simulink model "CAMFC2_01_WMR01"  (R2017b)
settings: Solver=ode45  StartTime=0.0  StopTime=150  RelTol=1e-3  EnableMultiTasking=on
InitFcn:
  | constant_CAMFC2_01_WMR01
values from neighbouring files (symbols this model uses):
  alpha = 0.1    [constant_CAMFC2_01_WMR01.m]    (also in constant_CAMFC2_04_Comp.m = 0.01; constant_CAMFC2_04_Quad_03.m; constant_CAMFC2_04_Simple.m = 0.01; constant_CAMFC2_04_Simple_DoubleIntegrator.m = 0.01)
  AN = [     0 1 0 0 ... (first row only)    [constant_CAMFC2_01_WMR01.m]    (also in constant_CAMFC2_04_Comp.m = [     0 1 0 0 1; constant_CAMFC2_04_Quad_03.m; constant_CAMFC2_04_Simple.m; constant_CAMFC2_04_Simple_DoubleIntegrator.m)
  B = eye(n)    [constant_CAMFC2_01_WMR01.m]    (also in constant_CAMFC2_04_Quad_03.m; constant_CAMFC2_Quad_New_02.m)
  B_pseudo_inverse = ((B'*B)^(-1))*B'    [constant_CAMFC2_01_WMR01.m]    (also in constant_CAMFC2_Quad_New_02.m)
  BN = [     1 0 0 0 ... (first row only)    [constant_CAMFC2_01_WMR01.m]    (also in constant_CAMFC2_04_Comp.m = [     0 0 0 0 0; constant_CAMFC2_04_Quad_03.m; constant_CAMFC2_04_Simple.m; constant_CAMFC2_04_Simple_DoubleIntegrator.m)
  chi = [0 0 0 0 ... (first row only)    [constant_CAMFC2_01_WMR01.m]    (also in constant_CAMFC2_04_Comp.m = X_m*ones(n0,1); constant_CAMFC2_04_Quad_03.m = X_m*ones(n0,1); constant_CAMFC2_04_Simple.m = X_m*ones(n0,1); constant_CAMFC2_04_Simple_DoubleIntegrator.m = X_m*ones(n0,1))
  Cv = 0.1    [constant_CAMFC2_01_WMR01.m]
  Cw = 0.1    [constant_CAMFC2_01_WMR01.m]
  epsilon_struct = struct('data',epsilon_InitVal)    [constant_CAMFC2_01_WMR01.m]    (also in constant_CAMFC2_04_Comp.m; constant_CAMFC2_04_Quad_03.m; constant_CAMFC2_04_Simple.m; constant_CAMFC2_04_Simple_DoubleIntegrator.m)
  gama1 = 1e4*diag([1e-6*ones(2,1);1e0*ones(2,1)])    [constant_CAMFC2_01_WMR01.m]    (also in constant_CAMFC2_04_Comp.m = 1e+3*diag([1e-6;1e-0]); constant_CAMFC2_04_Quad_03.m = 1e+2*diag(1e-0*ones(n0,1)); constant_CAMFC2_04_Simple.m = 1e+2*diag([1e-0;1e-0]); constant_CAMFC2_04_Simple_Formation.m = 1e+2*diag([1e-0;1e-0]))
  gama2 = 1e-2*diag([1e-6*ones(2,1);1e0*ones(2,1)])    [constant_CAMFC2_01_WMR01.m]    (also in constant_CAMFC2_04_Comp.m = 1e+0*diag([1e-6;1e-0]); constant_CAMFC2_04_Quad_03.m = 1e+0*diag(1e-0*ones(n0,1)); constant_CAMFC2_04_Simple.m = 1e+1*diag([1e-0;1e-0]); constant_CAMFC2_04_Simple_Formation.m = 1e+1*diag([1e-0;1e-0]))
  H = L + BN    [constant_CAMFC2_01_WMR01.m]    (also in constant_CAMFC2_04_Comp.m; constant_CAMFC2_04_Quad_03.m; constant_CAMFC2_04_Simple.m; constant_CAMFC2_04_Simple_DoubleIntegrator.m)
  J = 0.01    [constant_CAMFC2_01_WMR01.m]    (also in constant_CAMFC2_04_Quad_03.m = 1.0e-3 * diag([1 1 2],0); constant_CAMFC2_Quad_New_02.m = 1.2416e-3 * diag([1 1 2],0))
  K = 1e-2*eye(n)    [constant_CAMFC2_01_WMR01.m]    (also in constant_CAMFC2_Quad_New_02.m = 1e+1*eye(n))
  k1 = 1    [constant_CAMFC2_01_WMR01.m]    (also in constant_CAMFC2_04_Comp.m; constant_CAMFC2_04_Quad_03.m = 50; constant_CAMFC2_04_Simple.m; constant_CAMFC2_04_Simple_DoubleIntegrator.m)
  k2 = 1    [constant_CAMFC2_01_WMR01.m]    (also in constant_CAMFC2_04_Comp.m; constant_CAMFC2_04_Quad_03.m; constant_CAMFC2_04_Simple.m; constant_CAMFC2_04_Simple_DoubleIntegrator.m)
  L0 = 0.1    [constant_CAMFC2_01_WMR01.m]
  M = 1    [constant_CAMFC2_01_WMR01.m]    (also in constant_CAMFC2_04_Quad_03.m = 2; constant_CAMFC2_Quad_New_02.m = 2)
  N = 4    [constant_CAMFC2_01_WMR01.m]    (also in constant_CAMFC2_04_Comp.m = 5; constant_CAMFC2_04_Quad_03.m; constant_CAMFC2_04_Simple.m; constant_CAMFC2_04_Simple_DoubleIntegrator.m)
  n = 4    [constant_CAMFC2_01_WMR01.m]    (also in constant_CAMFC2_04_Comp.m = 2; constant_CAMFC2_04_Quad_03.m = 6; constant_CAMFC2_04_Simple.m = 2; constant_CAMFC2_04_Simple_DoubleIntegrator.m = 2)
  n0 = 2    [constant_CAMFC2_01_WMR01.m]    (also in constant_CAMFC2_04_Comp.m = 1; constant_CAMFC2_04_Quad_03.m = 3; constant_CAMFC2_04_Simple.m; constant_CAMFC2_04_Simple_DoubleIntegrator.m = 1)
  Observer_Gain = 100    [constant_CAMFC2_01_WMR01.m]    (also in constant_CAMFC2_04_Comp.m = 10; constant_CAMFC2_04_Quad_03.m = 1; constant_CAMFC2_04_Simple.m; constant_CAMFC2_04_Simple_DoubleIntegrator.m)
  Observer_Gain1 = 100    [constant_CAMFC2_01_WMR01.m]    (also in constant_CAMFC2_04_Comp.m = 10; constant_CAMFC2_04_Quad_03.m = 1; constant_CAMFC2_04_Simple.m; constant_CAMFC2_04_Simple_DoubleIntegrator.m)
  P_struct = struct('data',P_InitVal)    [constant_CAMFC2_01_WMR01.m]    (also in constant_CAMFC2_04_Comp.m; constant_CAMFC2_04_Quad_03.m; constant_CAMFC2_04_Simple.m; constant_CAMFC2_04_Simple_DoubleIntegrator.m)
  Q = 1e-0*eye(n)    [constant_CAMFC2_01_WMR01.m]    (also in constant_CAMFC2_04_Comp.m = 1.0e+2*eye(n); constant_CAMFC2_04_Quad_03.m = 1e-0*eye(n0); constant_CAMFC2_04_Simple.m = 1.0e+1*eye(n); constant_CAMFC2_04_Simple_Formation.m = 1.0e+1*eye(n))
  R = 1e-0*eye(n)    [constant_CAMFC2_01_WMR01.m]    (also in constant_CAMFC2_04_Quad_03.m; constant_CAMFC2_Quad_New_02.m = 1e+0*eye(n))
  R0 = 0.1    [constant_CAMFC2_01_WMR01.m]
  rho1 = 1e-1    (= 0.1)    [constant_CAMFC2_01_WMR01.m]    (also in constant_CAMFC2_04_Comp.m = 1; constant_CAMFC2_04_Quad_03.m = 1; constant_CAMFC2_04_Simple.m = 1; constant_CAMFC2_04_Simple_DoubleIntegrator.m = 1)
  rho2 = 1e-3    (= 0.001)    [constant_CAMFC2_01_WMR01.m]    (also in constant_CAMFC2_04_Comp.m = 1; constant_CAMFC2_04_Quad_03.m = 1; constant_CAMFC2_04_Simple.m = 1; constant_CAMFC2_04_Simple_DoubleIntegrator.m = 10)
  T_struct = struct('data',T_InitVal)    [constant_CAMFC2_01_WMR01.m]    (also in constant_CAMFC2_04_Comp.m; constant_CAMFC2_04_Quad_03.m; constant_CAMFC2_04_Simple.m; constant_CAMFC2_04_Simple_DoubleIntegrator.m)
  Thresh = 1e-4    (= 0.0001)    [constant_CAMFC2_01_WMR01.m]
  U_dot0_M = U_dot0_m*ones(n,1)    [constant_CAMFC2_01_WMR01.m]    (also in constant_CAMFC2_Quad_New_02.m = U_dot0_m*ones(n0,1))
  Upsilon_M = Upsilon_m*ones(n,1)    [constant_CAMFC2_01_WMR01.m]    (also in constant_CAMFC2_04_Comp.m; constant_CAMFC2_04_Quad_03.m = Upsilon_m*ones(n0,1); constant_CAMFC2_04_Simple.m; constant_CAMFC2_04_Simple_DoubleIntegrator.m)
libraries: simulink x1
(part 1 of 2)
settings Model: SimulationMode=rapid-accelerator  ExtModeTrigDuration=100  Creator=hp  LastModifiedBy=ali.safaei
settings DataIOCC: LimitDataPoints=on  SaveFinalState=on  SaveFormat=StructureWithTime  SaveOutput=off  SaveState=on  StateSaveName=tmp_raccel_xout  SignalLoggingName=tmp_raccel_logsout
settings OptimizationCC: EfficientMapNaN2IntZero=off  LifeSpan=inf
settings DebuggingCC: UnderspecifiedInitializationDetection=Classic  MergeDetectMultiDrivingBlocksExec=none  SFUnexpectedBacktrackingDiag=warning  SFNoUnconditionalDefaultTransitionDiag=warning  SFExecutionAtInitializationDiag=none
settings HardwareCC: ProdBitPerPointer=32  ProdBitPerSizeT=32  ProdBitPerPtrDiffT=32  ProdLargestAtomicFloat=None  ProdIntDivRoundTo=Undefined  ProdEndianess=Unspecified  ProdWordSize=32  ProdHWDeviceType=32-bit Generic  TargetBitPerPointer=64  TargetBitPerSizeT=64  TargetBitPerPtrDiffT=64  TargetLongLongMode=on  TargetIntDivRoundTo=Zero  TargetEndianess=LittleEndian  TargetWordSize=64  TargetHWDeviceType=MATLAB Host  ProdEqTarget=off
settings ModelReferenceCC: PropagateSignalLabelsOutOfModel=off
settings RTWCC: SystemTargetFile=raccel.tlc  TemplateMakefile=raccel_default_tmf  RTWVerbose=off  RTWUseSimCustomCode=on
settings CodeAppCC: GenerateComments=off  MaxIdLength=128  MangleLength=10  SimulinkBlockComments=off
settings RaccelTargetCC: GeneratePreprocessorConditionals=Use local settings  MultiInstanceERTCode=off  ExtModeMexArgs='', 0, 54523  ENABLE_SLEXEC_SSBRIDGE=0  RTWCAPIParams=on
settings ConfigComp: CovMetricSettings=dw  CovHtmlReporting=on  CovSaveCumulativeToWorkspaceVar=on  CovSaveSingleToWorkspaceVar=on  CovExternalEMLEnable=off

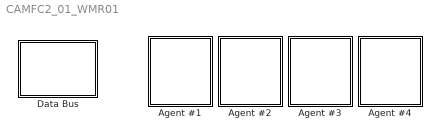
== system CAMFC2_01_WMR01 ==
  Agent #1 : Subsystem
  Agent #2 : Subsystem
  Agent #3 : Subsystem
  Agent #4 : Subsystem
  "Data Bus " : Subsystem

== system CAMFC2_01_WMR01/Agent #1 ==
  Agent # : Constant
  Controller interpreter : MATLAB Function  TreatAsAtomicUnit=on
  Decenteralized Cooperaive Controller #1 : Subsystem
  WMR Plant-01 : Subsystem
  tag scope: x1=global
  wires:
  Decenteralized Cooperaive Controller #1/1(U1) -> Controller interpreter/1(U)
  Agent #/1 -> Decenteralized Cooperaive Controller #1/1(Agent #)
  WMR Plant-01/1(Y) -> [x1]
  Controller interpreter/1(u) -> WMR Plant-01/1(U)

== system CAMFC2_01_WMR01/Agent #2 ==
  Agent # : Constant  Value=2
  Controller interpreter : MATLAB Function  TreatAsAtomicUnit=on
  Decenteralized Cooperaive Controller #2 : Subsystem
  WMR Plant-02 : Subsystem
  tag scope: x2=global
  wires:
  Agent #/1 -> Decenteralized Cooperaive Controller #2/1(Agent #)
  WMR Plant-02/1(Y) -> [x2]
  Decenteralized Cooperaive Controller #2/1(U2) -> Controller interpreter/1(U)
  Controller interpreter/1(u) -> WMR Plant-02/1(U)

== system CAMFC2_01_WMR01/Agent #3 ==
  Agent # : Constant  Value=3
  Controller interpreter : MATLAB Function  TreatAsAtomicUnit=on
  Decenteralized Cooperaive Controller #3 : Subsystem
  WMR Plant-03 : Subsystem
  tag scope: x3=global
  wires:
  Agent #/1 -> Decenteralized Cooperaive Controller #3/1(Agent #)
  WMR Plant-03/1(Y) -> [x3]
  Decenteralized Cooperaive Controller #3/1(U3) -> Controller interpreter/1(U)
  Controller interpreter/1(u) -> WMR Plant-03/1(U)

== system CAMFC2_01_WMR01/Agent #4 ==
  Agent # : Constant  Value=4
  Controller interpreter : MATLAB Function  TreatAsAtomicUnit=on
  Decenteralized Cooperaive Controller #4 : Subsystem
  WMR Plant-04 : Subsystem
  tag scope: x4=global
  wires:
  WMR Plant-04/1(Y) -> [x4]
  Agent #/1 -> Decenteralized Cooperaive Controller #4/1(Agent #)
  Decenteralized Cooperaive Controller #4/1(U4) -> Controller interpreter/1(U)
  Controller interpreter/1(u) -> WMR Plant-04/1(U)

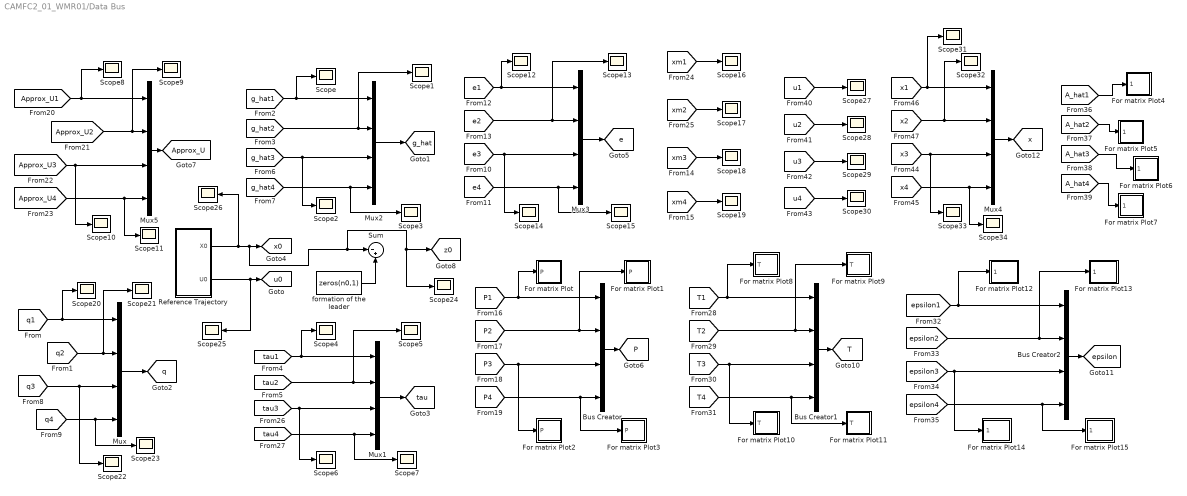
== system CAMFC2_01_WMR01/Data Bus  ==
  Bus Creator : BusCreator  Inputs=4  OutDataTypeStr=Bus: P_bus
  Bus Creator1 : BusCreator  Inputs=4  OutDataTypeStr=Bus: T_bus
  Bus Creator2 : BusCreator  Inputs=4  OutDataTypeStr=Bus: epsilon_bus
  For matrix Plot : Subsystem
  For matrix Plot1 : Subsystem
  For matrix Plot10 : Subsystem
  For matrix Plot11 : Subsystem
  For matrix Plot12 : Subsystem
  For matrix Plot13 : Subsystem
  For matrix Plot14 : Subsystem
  For matrix Plot15 : Subsystem
  For matrix Plot2 : Subsystem
  For matrix Plot3 : Subsystem
  For matrix Plot4 : Subsystem
  For matrix Plot5 : Subsystem
  For matrix Plot6 : Subsystem
  For matrix Plot7 : Subsystem
  For matrix Plot8 : Subsystem
  For matrix Plot9 : Subsystem
  Mux{,1..5} (6 alike) : Mux
  Reference Trajectory : Subsystem
  Scope{,1..34} (35 alike) : Scope
  Sum : Sum  Inputs=|-+
  formation of the leader : Constant  Value=zeros(n0,1)
  tag scope: Approx_U=global, P=global, T=global, e=global, epsilon=global, g_hat=global, q=global, tau=global, u0=global, x0=global, x=global, z0=global
  wires:
  [q2] -> Scope21/1, Mux/2
  [tau1] -> Scope4/1, Mux1/1
  [tau2] -> Scope5/1, Mux1/2
  Mux1/1 -> [tau]
  [q1] -> Scope20/1, Mux/1
  Reference Trajectory/2(U0) -> Scope25/1, [u0]
  [g_hat2] -> Mux2/2, Scope1/1
  Mux2/1 -> [g_hat]
  [g_hat1] -> Mux2/1, Scope/1
  Mux/1 -> [q]
  [e2] -> Scope13/1, Mux3/2
  [e1] -> Scope12/1, Mux3/1
  Mux3/1 -> [e]
  [P2] -> For matrix Plot1/1(P), Bus Creator/2
  [P1] -> For matrix Plot/1(P), Bus Creator/1
  Bus Creator/1 -> [P]
  [Approx_U2] -> Scope9/1, Mux5/2
  [Approx_U1] -> Mux5/1, Scope8/1
  Mux5/1 -> [Approx_U]
  Reference Trajectory/1(X0) -> Scope26/1, Scope24/1, [z0], Sum/1, [x0]
  [xm2] -> Scope17/1
  [xm1] -> Scope16/1
  [g_hat3] -> Scope2/1, Mux2/3
  [g_hat4] -> Scope3/1, Mux2/4
  [q4] -> Scope23/1, Mux/4
  [q3] -> Scope22/1, Mux/3
  [e3] -> Scope14/1, Mux3/3
  [e4] -> Scope15/1, Mux3/4
  [xm3] -> Scope18/1
  [xm4] -> Scope19/1
  [P3] -> For matrix Plot2/1(P), Bus Creator/3
  [P4] -> For matrix Plot3/1(P), Bus Creator/4
  [Approx_U3] -> Scope10/1, Mux5/3
  [Approx_U4] -> Scope11/1, Mux5/4
  [tau3] -> Scope6/1, Mux1/3
  [tau4] -> Scope7/1, Mux1/4
  [T2] -> For matrix Plot9/1(T), Bus Creator1/2
  [T1] -> For matrix Plot8/1(T), Bus Creator1/1
  Bus Creator1/1 -> [T]
  [T3] -> For matrix Plot10/1(T), Bus Creator1/3
  [T4] -> For matrix Plot11/1(T), Bus Creator1/4
  [epsilon2] -> For matrix Plot13/1(epsilon), Bus Creator2/2
  [epsilon1] -> For matrix Plot12/1(epsilon), Bus Creator2/1
  Bus Creator2/1 -> [epsilon]
  [epsilon3] -> For matrix Plot14/1(epsilon), Bus Creator2/3
  [epsilon4] -> For matrix Plot15/1(epsilon), Bus Creator2/4
  [A_hat2] -> For matrix Plot5/1(A_hat)
  [A_hat1] -> For matrix Plot4/1(A_hat)
  [A_hat3] -> For matrix Plot6/1(A_hat)
  [A_hat4] -> For matrix Plot7/1(A_hat)
  [u2] -> Scope28/1
  [u1] -> Scope27/1
  [u4] -> Scope30/1
  [u3] -> Scope29/1
  formation of the leader/1 -> Sum/2
  [x4] -> Mux4/4, Scope34/1
  [x3] -> Mux4/3, Scope33/1
  Mux4/1 -> [x]
  [x1] -> Mux4/1, Scope31/1
  [x2] -> Mux4/2, Scope32/1

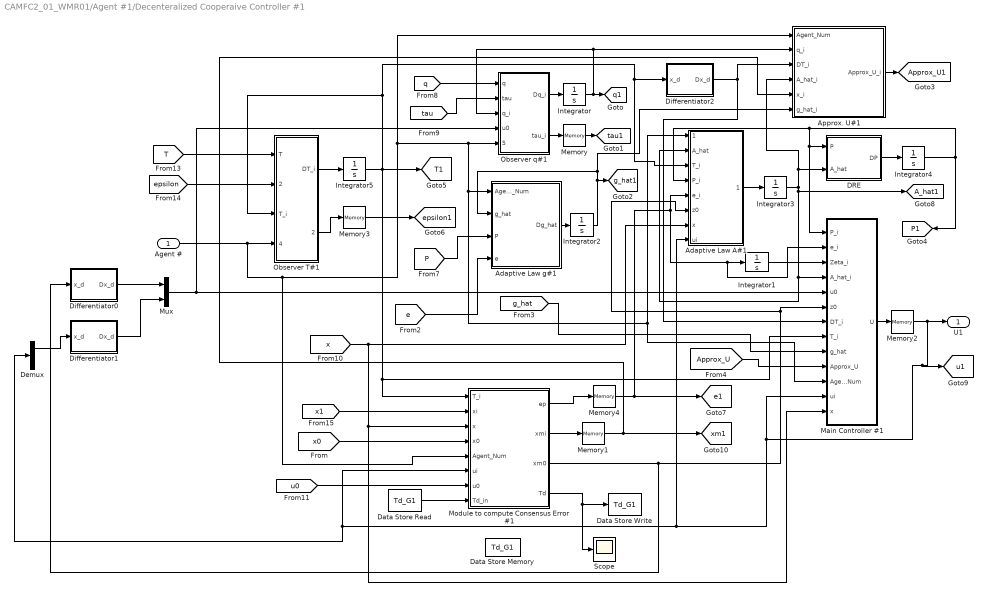
== system CAMFC2_01_WMR01/Agent #1/Decenteralized Cooperaive Controller #1 ==
  Agent # : Inport
  Adaptive Law A#1 : MATLAB Function  TreatAsAtomicUnit=on
  Adaptive Law g#1 : MATLAB Function  TreatAsAtomicUnit=on
  Approx. U#1 : MATLAB Function  TreatAsAtomicUnit=on
  DRE : MATLAB Function  TreatAsAtomicUnit=on
  Data Store Memory : DataStoreMemory  DataStoreName=Td_G1  ReadBeforeWriteMsg=warning  WriteAfterWriteMsg=warning  WriteAfterReadMsg=warning  VectorParams1D=off  ShowAdditionalParam=off
  Data Store Read : DataStoreRead  DataStoreName=Td_G1
  Data Store Write : DataStoreWrite  DataStoreName=Td_G1
  Demux : Demux  Outputs=2
  Differentiator0 : Subsystem
  Differentiator1 : Subsystem
  Differentiator2 : Subsystem
  Integrator : Integrator  InitialCondition=zeros(n,1)
  Integrator1 : Integrator  InitialCondition=zeros(n,1)
  Integrator2 : Integrator  InitialCondition=zeros(n,1)
  Integrator3 : Integrator  InitialCondition=zeros(n)
  Integrator4 : Integrator  InitialCondition=eye(n)
  Integrator5 : Integrator  InitialCondition=zeros(N+1,n)
  Main Controller #1 : MATLAB Function  TreatAsAtomicUnit=on
  Memory{,1..2,4} (4 alike) : Memory  InitialCondition=zeros(n,1)
  Memory3 : Memory  InitialCondition=zeros(N+1,n)
  Module to compute Consensus Error #1 : MATLAB Function  TreatAsAtomicUnit=on
  Mux : Mux  Inputs=2
  Observer T#1 : MATLAB Function  TreatAsAtomicUnit=on
  Observer q#1 : MATLAB Function  TreatAsAtomicUnit=on
  Scope : Scope
  U1 : Outport
  tag scope: A_hat1=global, Approx_U1=global, P1=global, T1=global, e1=global, epsilon1=global, g_hat1=global, q1=global, tau1=global, u1=global, xm1=global
  wires:
  [x] -> Adaptive Law A#1/7(x), Main Controller #1/13(x), Module to compute Consensus Error #1/3(x)
  Module to compute Consensus Error #1/1(ep) -> Memory4/1
  Differentiator2/1(Dx_d) -> Main Controller #1/7(DT_i), Approx. U#1/3(DT_i)
  Integrator1/1 -> Main Controller #1/3(Zeta_i)
  [epsilon] -> Observer T#1/2(epsilon)
  [T] -> Observer T#1/1(T)
  Memory3/1 -> [epsilon1]
  Observer T#1/2(epsilon_i) -> Memory3/1
  Integrator5/1 -> Main Controller #1/8(T_i), Module to compute Consensus Error #1/1(T_i), [T1], Adaptive Law A#1/3(T_i), Differentiator2/1(x_d), Observer T#1/3(T_i)
  Observer T#1/1(DT_i) -> Integrator5/1
  Memory4/1 -> [e1], Adaptive Law A#1/5(e_i), Main Controller #1/2(e_i), Integrator1/1
  Integrator3/1 -> Approx. U#1/4(A_hat_i), DRE/2(A_hat), [A_hat1], Adaptive Law A#1/2(A_hat), Main Controller #1/4(A_hat_i)
  [tau] -> Observer q#1/2(tau)
  [q] -> Observer q#1/1(q)
  [e] -> Adaptive Law g#1/4(e)
  [P] -> Adaptive Law g#1/3(P)
  Integrator4/1 -> [P1], Adaptive Law A#1/4(P_i), DRE/1(P), Main Controller #1/1(P_i)
  [g_hat] -> Main Controller #1/9(g_hat)
  [Approx_U] -> Main Controller #1/10(Approx_U)
  Integrator/1 -> [q1], Observer q#1/3(q_i), Approx. U#1/2(q_i)
  Integrator2/1 -> [g_hat1], Adaptive Law g#1/2(g_hat), Approx. U#1/6(g_hat_i)
  Adaptive Law g#1/1(Dg_hat) -> Integrator2/1
  Observer q#1/2(tau_i) -> Memory/1
  Observer q#1/1(Dq_i) -> Integrator/1
  Agent #/1 -> Observer T#1/4(Agent_Num), Module to compute Consensus Error #1/5(Agent_Num), Approx. U#1/1(Agent_Num), Adaptive Law g#1/1(Agent_Num), Main Controller #1/11(Agent_Num), Adaptive Law A#1/1(Agent_Num), Observer q#1/5(Agent_Num)
  Memory/1 -> [tau1]
  Approx. U#1/1(Approx_U_i) -> [Approx_U1]
  Memory2/1 -> U1/1, Module to compute Consensus Error #1/6(ui), Demux/1, Adaptive Law A#1/8(ui), Main Controller #1/12(ui), [u1]
  DRE/1(DP) -> Integrator4/1
  Main Controller #1/1(U) -> Memory2/1
  Adaptive Law A#1/1(DA_hat) -> Integrator3/1
  Mux/1 -> Main Controller #1/5(u0), Observer q#1/4(u0)
  Demux/1 -> Differentiator1/1(x_d)
  [x1] -> Module to compute Consensus Error #1/2(xi)
  [x0] -> Module to compute Consensus Error #1/4(x0)
  [u0] -> Module to compute Consensus Error #1/7(u0)
  Differentiator0/1(Dx_d) -> Mux/1
  Differentiator1/1(Dx_d) -> Mux/2
  Module to compute Consensus Error #1/2(xmi) -> Memory1/1
  Module to compute Consensus Error #1/4(Td) -> Scope/1, Data Store Write/1
  Data Store Read/1 -> Module to compute Consensus Error #1/8(Td_in)
  Memory1/1 -> [xm1], Approx. U#1/5(x_i)
  Module to compute Consensus Error #1/3(xm0) -> Differentiator0/1(x_d), Main Controller #1/6(z0), Adaptive Law A#1/6(z0)

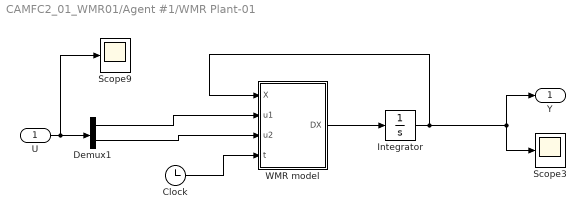
== system CAMFC2_01_WMR01/Agent #1/WMR Plant-01 ==
  U : Inport
  Clock : Clock
  Demux1 : Demux  Outputs=2
  Integrator : Integrator  InitialCondition=[0;0;0;0;0]
  Scope3 : Scope
  Scope9 : Scope
  WMR model : MATLAB Function  TreatAsAtomicUnit=on
  Y : Outport
  wires:
  Integrator/1 -> WMR model/1(X), Y/1, Scope3/1
  WMR model/1(DX) -> Integrator/1
  U/1 -> Scope9/1, Demux1/1
  Demux1/1 -> WMR model/2(u1)
  Demux1/2 -> WMR model/3(u2)
  Clock/1 -> WMR model/4(t)

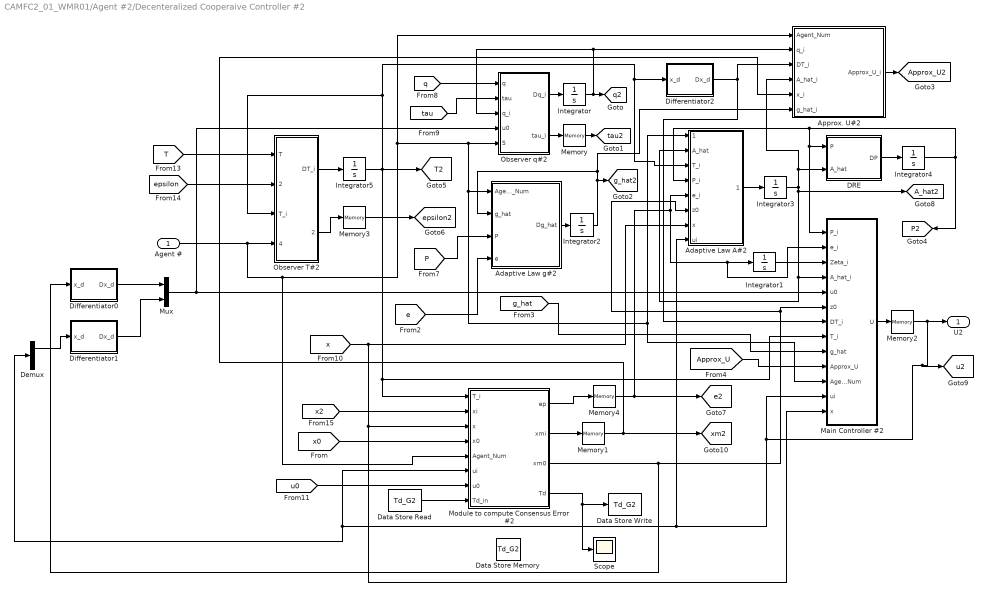
== system CAMFC2_01_WMR01/Agent #2/Decenteralized Cooperaive Controller #2 ==
  Agent # : Inport
  Adaptive Law A#2 : MATLAB Function  TreatAsAtomicUnit=on
  Adaptive Law g#2 : MATLAB Function  TreatAsAtomicUnit=on
  Approx. U#2 : MATLAB Function  TreatAsAtomicUnit=on
  DRE : MATLAB Function  TreatAsAtomicUnit=on
  Data Store Memory : DataStoreMemory  DataStoreName=Td_G2  ReadBeforeWriteMsg=warning  WriteAfterWriteMsg=warning  WriteAfterReadMsg=warning  VectorParams1D=off  ShowAdditionalParam=off
  Data Store Read : DataStoreRead  DataStoreName=Td_G2
  Data Store Write : DataStoreWrite  DataStoreName=Td_G2
  Demux : Demux  Outputs=2
  Differentiator0 : Subsystem
  Differentiator1 : Subsystem
  Differentiator2 : Subsystem
  Integrator : Integrator  InitialCondition=zeros(n,1)
  Integrator1 : Integrator  InitialCondition=zeros(n,1)
  Integrator2 : Integrator  InitialCondition=zeros(n,1)
  Integrator3 : Integrator  InitialCondition=zeros(n)
  Integrator4 : Integrator  InitialCondition=eye(n)
  Integrator5 : Integrator  InitialCondition=zeros(N+1,n)
  Main Controller #2 : MATLAB Function  TreatAsAtomicUnit=on
  Memory{,1..2,4} (4 alike) : Memory  InitialCondition=zeros(n,1)
  Memory3 : Memory  InitialCondition=zeros(N+1,n)
  Module to compute Consensus Error #2 : MATLAB Function  TreatAsAtomicUnit=on
  Mux : Mux  Inputs=2
  Observer T#2 : MATLAB Function  TreatAsAtomicUnit=on
  Observer q#2 : MATLAB Function  TreatAsAtomicUnit=on
  Scope : Scope
  U2 : Outport
  tag scope: A_hat2=global, Approx_U2=global, P2=global, T2=global, e2=global, epsilon2=global, g_hat2=global, q2=global, tau2=global, u2=global, xm2=global
  wires:
  [x] -> Adaptive Law A#2/7(x), Main Controller #2/13(x), Module to compute Consensus Error #2/3(x)
  Module to compute Consensus Error #2/1(ep) -> Memory4/1
  Differentiator2/1(Dx_d) -> Main Controller #2/7(DT_i), Approx. U#2/3(DT_i)
  Integrator1/1 -> Main Controller #2/3(Zeta_i)
  [epsilon] -> Observer T#2/2(epsilon)
  [T] -> Observer T#2/1(T)
  Memory3/1 -> [epsilon2]
  Observer T#2/2(epsilon_i) -> Memory3/1
  Integrator5/1 -> Main Controller #2/8(T_i), Module to compute Consensus Error #2/1(T_i), [T2], Adaptive Law A#2/3(T_i), Differentiator2/1(x_d), Observer T#2/3(T_i)
  Observer T#2/1(DT_i) -> Integrator5/1
  Memory4/1 -> [e2], Adaptive Law A#2/5(e_i), Main Controller #2/2(e_i), Integrator1/1
  Integrator3/1 -> Approx. U#2/4(A_hat_i), DRE/2(A_hat), [A_hat2], Adaptive Law A#2/2(A_hat), Main Controller #2/4(A_hat_i)
  [tau] -> Observer q#2/2(tau)
  [q] -> Observer q#2/1(q)
  [e] -> Adaptive Law g#2/4(e)
  [P] -> Adaptive Law g#2/3(P)
  Integrator4/1 -> [P2], Adaptive Law A#2/4(P_i), DRE/1(P), Main Controller #2/1(P_i)
  [g_hat] -> Main Controller #2/9(g_hat)
  [Approx_U] -> Main Controller #2/10(Approx_U)
  Integrator/1 -> [q2], Observer q#2/3(q_i), Approx. U#2/2(q_i)
  Integrator2/1 -> [g_hat2], Adaptive Law g#2/2(g_hat), Approx. U#2/6(g_hat_i)
  Adaptive Law g#2/1(Dg_hat) -> Integrator2/1
  Observer q#2/2(tau_i) -> Memory/1
  Observer q#2/1(Dq_i) -> Integrator/1
  Agent #/1 -> Observer T#2/4(Agent_Num), Module to compute Consensus Error #2/5(Agent_Num), Approx. U#2/1(Agent_Num), Adaptive Law g#2/1(Agent_Num), Main Controller #2/11(Agent_Num), Adaptive Law A#2/1(Agent_Num), Observer q#2/5(Agent_Num)
  Memory/1 -> [tau2]
  Approx. U#2/1(Approx_U_i) -> [Approx_U2]
  Memory2/1 -> U2/1, Module to compute Consensus Error #2/6(ui), Demux/1, Adaptive Law A#2/8(ui), Main Controller #2/12(ui), [u2]
  DRE/1(DP) -> Integrator4/1
  Main Controller #2/1(U) -> Memory2/1
  Adaptive Law A#2/1(DA_hat) -> Integrator3/1
  Mux/1 -> Main Controller #2/5(u0), Observer q#2/4(u0)
  Demux/1 -> Differentiator1/1(x_d)
  [x2] -> Module to compute Consensus Error #2/2(xi)
  [x0] -> Module to compute Consensus Error #2/4(x0)
  [u0] -> Module to compute Consensus Error #2/7(u0)
  Differentiator0/1(Dx_d) -> Mux/1
  Differentiator1/1(Dx_d) -> Mux/2
  Module to compute Consensus Error #2/2(xmi) -> Memory1/1
  Module to compute Consensus Error #2/4(Td) -> Scope/1, Data Store Write/1
  Data Store Read/1 -> Module to compute Consensus Error #2/8(Td_in)
  Memory1/1 -> [xm2], Approx. U#2/5(x_i)
  Module to compute Consensus Error #2/3(xm0) -> Differentiator0/1(x_d), Main Controller #2/6(z0), Adaptive Law A#2/6(z0)

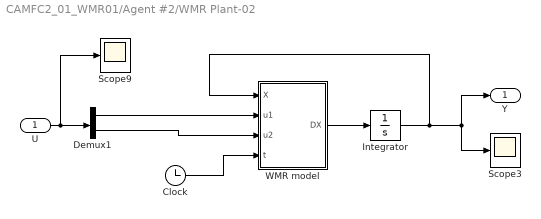
== system CAMFC2_01_WMR01/Agent #2/WMR Plant-02 ==
  U : Inport
  Clock : Clock
  Demux1 : Demux  Outputs=2
  Integrator : Integrator  InitialCondition=[0;0;0;0;0]
  Scope3 : Scope
  Scope9 : Scope
  WMR model : MATLAB Function  TreatAsAtomicUnit=on
  Y : Outport
  wires:
  Integrator/1 -> WMR model/1(X), Y/1, Scope3/1
  WMR model/1(DX) -> Integrator/1
  U/1 -> Scope9/1, Demux1/1
  Demux1/1 -> WMR model/2(u1)
  Demux1/2 -> WMR model/3(u2)
  Clock/1 -> WMR model/4(t)

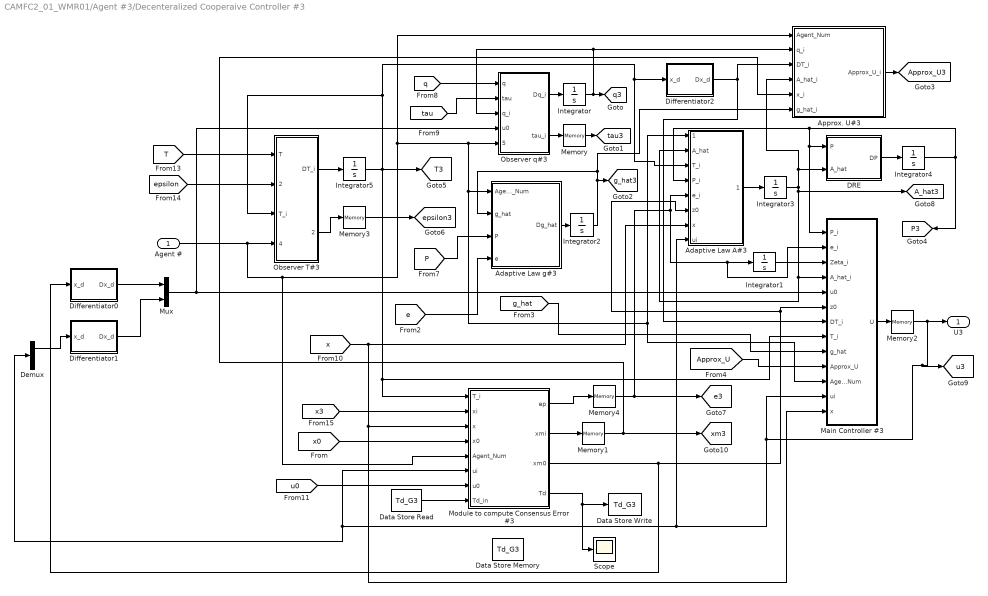
== system CAMFC2_01_WMR01/Agent #3/Decenteralized Cooperaive Controller #3 ==
  Agent # : Inport
  Adaptive Law A#3 : MATLAB Function  TreatAsAtomicUnit=on
  Adaptive Law g#3 : MATLAB Function  TreatAsAtomicUnit=on
  Approx. U#3 : MATLAB Function  TreatAsAtomicUnit=on
  DRE : MATLAB Function  TreatAsAtomicUnit=on
  Data Store Memory : DataStoreMemory  DataStoreName=Td_G3  ReadBeforeWriteMsg=warning  WriteAfterWriteMsg=warning  WriteAfterReadMsg=warning  VectorParams1D=off  ShowAdditionalParam=off
  Data Store Read : DataStoreRead  DataStoreName=Td_G3
  Data Store Write : DataStoreWrite  DataStoreName=Td_G3
  Demux : Demux  Outputs=2
  Differentiator0 : Subsystem
  Differentiator1 : Subsystem
  Differentiator2 : Subsystem
  Integrator : Integrator  InitialCondition=zeros(n,1)
  Integrator1 : Integrator  InitialCondition=zeros(n,1)
  Integrator2 : Integrator  InitialCondition=zeros(n,1)
  Integrator3 : Integrator  InitialCondition=zeros(n)
  Integrator4 : Integrator  InitialCondition=eye(n)
  Integrator5 : Integrator  InitialCondition=zeros(N+1,n)
  Main Controller #3 : MATLAB Function  TreatAsAtomicUnit=on
  Memory{,1..2,4} (4 alike) : Memory  InitialCondition=zeros(n,1)
  Memory3 : Memory  InitialCondition=zeros(N+1,n)
  Module to compute Consensus Error #3 : MATLAB Function  TreatAsAtomicUnit=on
  Mux : Mux  Inputs=2
  Observer T#3 : MATLAB Function  TreatAsAtomicUnit=on
  Observer q#3 : MATLAB Function  TreatAsAtomicUnit=on
  Scope : Scope
  U3 : Outport
  tag scope: A_hat3=global, Approx_U3=global, P3=global, T3=global, e3=global, epsilon3=global, g_hat3=global, q3=global, tau3=global, u3=global, xm3=global
  wires:
  [x] -> Adaptive Law A#3/7(x), Main Controller #3/13(x), Module to compute Consensus Error #3/3(x)
  Module to compute Consensus Error #3/1(ep) -> Memory4/1
  Differentiator2/1(Dx_d) -> Main Controller #3/7(DT_i), Approx. U#3/3(DT_i)
  Integrator1/1 -> Main Controller #3/3(Zeta_i)
  [epsilon] -> Observer T#3/2(epsilon)
  [T] -> Observer T#3/1(T)
  Memory3/1 -> [epsilon3]
  Observer T#3/2(epsilon_i) -> Memory3/1
  Integrator5/1 -> Main Controller #3/8(T_i), Module to compute Consensus Error #3/1(T_i), [T3], Adaptive Law A#3/3(T_i), Differentiator2/1(x_d), Observer T#3/3(T_i)
  Observer T#3/1(DT_i) -> Integrator5/1
  Memory4/1 -> [e3], Adaptive Law A#3/5(e_i), Main Controller #3/2(e_i), Integrator1/1
  Integrator3/1 -> Approx. U#3/4(A_hat_i), DRE/2(A_hat), [A_hat3], Adaptive Law A#3/2(A_hat), Main Controller #3/4(A_hat_i)
  [tau] -> Observer q#3/2(tau)
  [q] -> Observer q#3/1(q)
  [e] -> Adaptive Law g#3/4(e)
  [P] -> Adaptive Law g#3/3(P)
  Integrator4/1 -> [P3], Adaptive Law A#3/4(P_i), DRE/1(P), Main Controller #3/1(P_i)
  [g_hat] -> Main Controller #3/9(g_hat)
  [Approx_U] -> Main Controller #3/10(Approx_U)
  Integrator/1 -> [q3], Observer q#3/3(q_i), Approx. U#3/2(q_i)
  Integrator2/1 -> [g_hat3], Adaptive Law g#3/2(g_hat), Approx. U#3/6(g_hat_i)
  Adaptive Law g#3/1(Dg_hat) -> Integrator2/1
  Observer q#3/2(tau_i) -> Memory/1
  Observer q#3/1(Dq_i) -> Integrator/1
  Agent #/1 -> Observer T#3/4(Agent_Num), Module to compute Consensus Error #3/5(Agent_Num), Approx. U#3/1(Agent_Num), Adaptive Law g#3/1(Agent_Num), Main Controller #3/11(Agent_Num), Adaptive Law A#3/1(Agent_Num), Observer q#3/5(Agent_Num)
  Memory/1 -> [tau3]
  Approx. U#3/1(Approx_U_i) -> [Approx_U3]
  Memory2/1 -> U3/1, Module to compute Consensus Error #3/6(ui), Demux/1, Adaptive Law A#3/8(ui), Main Controller #3/12(ui), [u3]
  DRE/1(DP) -> Integrator4/1
  Main Controller #3/1(U) -> Memory2/1
  Adaptive Law A#3/1(DA_hat) -> Integrator3/1
  Mux/1 -> Main Controller #3/5(u0), Observer q#3/4(u0)
  Demux/1 -> Differentiator1/1(x_d)
  [x3] -> Module to compute Consensus Error #3/2(xi)
  [x0] -> Module to compute Consensus Error #3/4(x0)
  [u0] -> Module to compute Consensus Error #3/7(u0)
  Differentiator0/1(Dx_d) -> Mux/1
  Differentiator1/1(Dx_d) -> Mux/2
  Module to compute Consensus Error #3/2(xmi) -> Memory1/1
  Module to compute Consensus Error #3/4(Td) -> Scope/1, Data Store Write/1
  Data Store Read/1 -> Module to compute Consensus Error #3/8(Td_in)
  Memory1/1 -> [xm3], Approx. U#3/5(x_i)
  Module to compute Consensus Error #3/3(xm0) -> Differentiator0/1(x_d), Main Controller #3/6(z0), Adaptive Law A#3/6(z0)

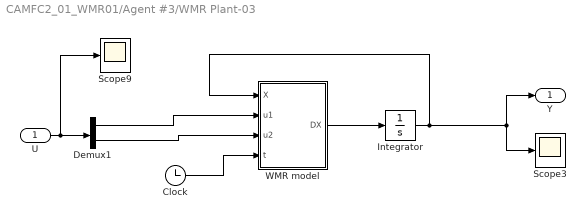
== system CAMFC2_01_WMR01/Agent #3/WMR Plant-03 ==
  U : Inport
  Clock : Clock
  Demux1 : Demux  Outputs=2
  Integrator : Integrator  InitialCondition=[0;0;0;0;0]
  Scope3 : Scope
  Scope9 : Scope
  WMR model : MATLAB Function  TreatAsAtomicUnit=on
  Y : Outport
  wires:
  Integrator/1 -> WMR model/1(X), Y/1, Scope3/1
  WMR model/1(DX) -> Integrator/1
  U/1 -> Scope9/1, Demux1/1
  Demux1/1 -> WMR model/2(u1)
  Demux1/2 -> WMR model/3(u2)
  Clock/1 -> WMR model/4(t)

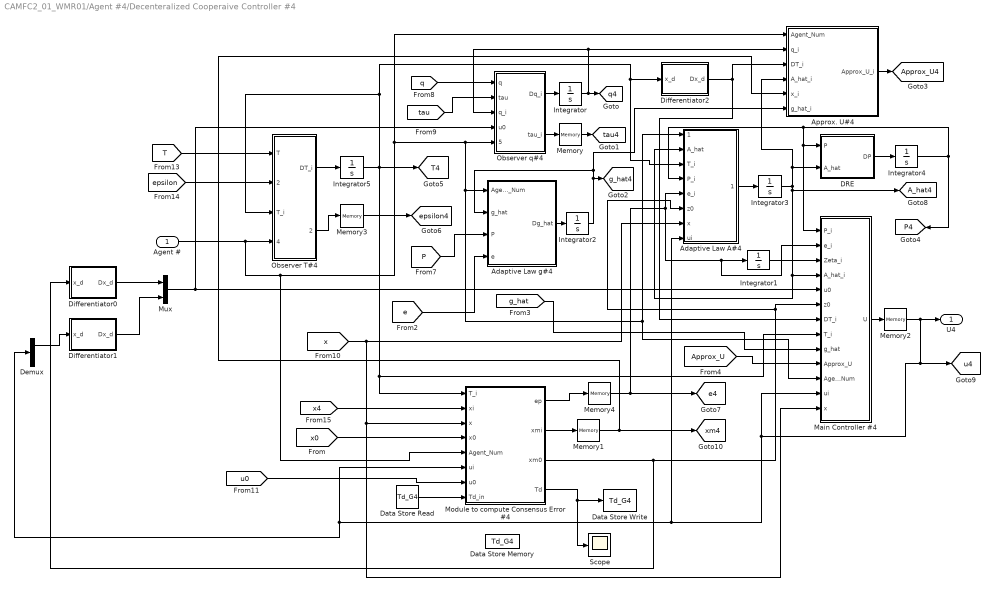
== system CAMFC2_01_WMR01/Agent #4/Decenteralized Cooperaive Controller #4 ==
  Agent # : Inport
  Adaptive Law A#4 : MATLAB Function  TreatAsAtomicUnit=on
  Adaptive Law g#4 : MATLAB Function  TreatAsAtomicUnit=on
  Approx. U#4 : MATLAB Function  TreatAsAtomicUnit=on
  DRE : MATLAB Function  TreatAsAtomicUnit=on
  Data Store Memory : DataStoreMemory  DataStoreName=Td_G4  ReadBeforeWriteMsg=warning  WriteAfterWriteMsg=warning  WriteAfterReadMsg=warning  VectorParams1D=off  ShowAdditionalParam=off
  Data Store Read : DataStoreRead  DataStoreName=Td_G4
  Data Store Write : DataStoreWrite  DataStoreName=Td_G4
  Demux : Demux  Outputs=2
  Differentiator0 : Subsystem
  Differentiator1 : Subsystem
  Differentiator2 : Subsystem
  Integrator : Integrator  InitialCondition=zeros(n,1)
  Integrator1 : Integrator  InitialCondition=zeros(n,1)
  Integrator2 : Integrator  InitialCondition=zeros(n,1)
  Integrator3 : Integrator  InitialCondition=zeros(n)
  Integrator4 : Integrator  InitialCondition=eye(n)
  Integrator5 : Integrator  InitialCondition=zeros(N+1,n)
  Main Controller #4 : MATLAB Function  TreatAsAtomicUnit=on
  Memory{,1..2,4} (4 alike) : Memory  InitialCondition=zeros(n,1)
  Memory3 : Memory  InitialCondition=zeros(N+1,n)
  Module to compute Consensus Error #4 : MATLAB Function  TreatAsAtomicUnit=on
  Mux : Mux  Inputs=2
  Observer T#4 : MATLAB Function  TreatAsAtomicUnit=on
  Observer q#4 : MATLAB Function  TreatAsAtomicUnit=on
  Scope : Scope
  U4 : Outport
  tag scope: A_hat4=global, Approx_U4=global, P4=global, T4=global, e4=global, epsilon4=global, g_hat4=global, q4=global, tau4=global, u4=global, xm4=global
  wires:
  [x] -> Adaptive Law A#4/7(x), Main Controller #4/13(x), Module to compute Consensus Error #4/3(x)
  Module to compute Consensus Error #4/1(ep) -> Memory4/1
  Differentiator2/1(Dx_d) -> Main Controller #4/7(DT_i), Approx. U#4/3(DT_i)
  Integrator1/1 -> Main Controller #4/3(Zeta_i)
  [epsilon] -> Observer T#4/2(epsilon)
  [T] -> Observer T#4/1(T)
  Memory3/1 -> [epsilon4]
  Observer T#4/2(epsilon_i) -> Memory3/1
  Integrator5/1 -> Main Controller #4/8(T_i), Module to compute Consensus Error #4/1(T_i), [T4], Adaptive Law A#4/3(T_i), Differentiator2/1(x_d), Observer T#4/3(T_i)
  Observer T#4/1(DT_i) -> Integrator5/1
  Memory4/1 -> [e4], Adaptive Law A#4/5(e_i), Main Controller #4/2(e_i), Integrator1/1
  Integrator3/1 -> Approx. U#4/4(A_hat_i), DRE/2(A_hat), [A_hat4], Adaptive Law A#4/2(A_hat), Main Controller #4/4(A_hat_i)
  [tau] -> Observer q#4/2(tau)
  [q] -> Observer q#4/1(q)
  [e] -> Adaptive Law g#4/4(e)
  [P] -> Adaptive Law g#4/3(P)
  Integrator4/1 -> [P4], Adaptive Law A#4/4(P_i), DRE/1(P), Main Controller #4/1(P_i)
  [g_hat] -> Main Controller #4/9(g_hat)
  [Approx_U] -> Main Controller #4/10(Approx_U)
  Integrator/1 -> [q4], Observer q#4/3(q_i), Approx. U#4/2(q_i)
  Integrator2/1 -> [g_hat4], Adaptive Law g#4/2(g_hat), Approx. U#4/6(g_hat_i)
  Adaptive Law g#4/1(Dg_hat) -> Integrator2/1
  Observer q#4/2(tau_i) -> Memory/1
  Observer q#4/1(Dq_i) -> Integrator/1
  Agent #/1 -> Observer T#4/4(Agent_Num), Module to compute Consensus Error #4/5(Agent_Num), Approx. U#4/1(Agent_Num), Adaptive Law g#4/1(Agent_Num), Main Controller #4/11(Agent_Num), Adaptive Law A#4/1(Agent_Num), Observer q#4/5(Agent_Num)
  Memory/1 -> [tau4]
  Approx. U#4/1(Approx_U_i) -> [Approx_U4]
  Memory2/1 -> U4/1, Module to compute Consensus Error #4/6(ui), Demux/1, Adaptive Law A#4/8(ui), Main Controller #4/12(ui), [u4]
  DRE/1(DP) -> Integrator4/1
  Main Controller #4/1(U) -> Memory2/1
  Adaptive Law A#4/1(DA_hat) -> Integrator3/1
  Mux/1 -> Main Controller #4/5(u0), Observer q#4/4(u0)
  Demux/1 -> Differentiator1/1(x_d)
  [x4] -> Module to compute Consensus Error #4/2(xi)
  [x0] -> Module to compute Consensus Error #4/4(x0)
  [u0] -> Module to compute Consensus Error #4/7(u0)
  Differentiator0/1(Dx_d) -> Mux/1
  Differentiator1/1(Dx_d) -> Mux/2
  Module to compute Consensus Error #4/2(xmi) -> Memory1/1
  Module to compute Consensus Error #4/4(Td) -> Scope/1, Data Store Write/1
  Data Store Read/1 -> Module to compute Consensus Error #4/8(Td_in)
  Memory1/1 -> [xm4], Approx. U#4/5(x_i)
  Module to compute Consensus Error #4/3(xm0) -> Differentiator0/1(x_d), Main Controller #4/6(z0), Adaptive Law A#4/6(z0)

== system CAMFC2_01_WMR01/Agent #4/WMR Plant-04 ==
  U : Inport
  Clock : Clock
  Demux1 : Demux  Outputs=2
  Integrator : Integrator  InitialCondition=[0;0;0;0;0]
  Scope3 : Scope
  Scope9 : Scope
  WMR model : MATLAB Function  TreatAsAtomicUnit=on
  Y : Outport
  wires:
  Integrator/1 -> WMR model/1(X), Y/1, Scope3/1
  WMR model/1(DX) -> Integrator/1
  U/1 -> Scope9/1, Demux1/1
  Demux1/1 -> WMR model/2(u1)
  Demux1/2 -> WMR model/3(u2)
  Clock/1 -> WMR model/4(t)

== system CAMFC2_01_WMR01/Data Bus /For matrix Plot ==
  P : Inport
  MATLAB Function : MATLAB Function  TreatAsAtomicUnit=on
  Scope24 : Scope
  To Workspace : ToWorkspace  VariableName=P1  SaveFormat=Structure With Time  SampleTime=-1
  wires:
  P/1 -> MATLAB Function/1(u)
  MATLAB Function/1(y) -> Scope24/1, To Workspace/1

== system CAMFC2_01_WMR01/Data Bus /For matrix Plot1 ==
  P : Inport
  MATLAB Function : MATLAB Function  TreatAsAtomicUnit=on
  Scope24 : Scope
  To Workspace : ToWorkspace  VariableName=P2  SaveFormat=Structure With Time  SampleTime=-1
  wires:
  MATLAB Function/1(y) -> Scope24/1, To Workspace/1
  P/1 -> MATLAB Function/1(u)

== system CAMFC2_01_WMR01/Data Bus /For matrix Plot10 ==
  T : Inport
  MATLAB Function : MATLAB Function  TreatAsAtomicUnit=on
  Scope24 : Scope
  To Workspace : ToWorkspace  VariableName=T3  SaveFormat=Structure With Time  SampleTime=-1
  wires:
  T/1 -> MATLAB Function/1(u)
  MATLAB Function/1(y) -> Scope24/1, To Workspace/1

== system CAMFC2_01_WMR01/Data Bus /For matrix Plot11 ==
  T : Inport
  MATLAB Function : MATLAB Function  TreatAsAtomicUnit=on
  Scope24 : Scope
  To Workspace : ToWorkspace  VariableName=T4  SaveFormat=Structure With Time  SampleTime=-1
  wires:
  MATLAB Function/1(y) -> Scope24/1, To Workspace/1
  T/1 -> MATLAB Function/1(u)

== system CAMFC2_01_WMR01/Data Bus /For matrix Plot12 ==
  epsilon : Inport
  MATLAB Function : MATLAB Function  TreatAsAtomicUnit=on
  Scope24 : Scope
  To Workspace : ToWorkspace  VariableName=epsilon1  SaveFormat=Structure With Time  SampleTime=-1
  wires:
  epsilon/1 -> MATLAB Function/1(u)
  MATLAB Function/1(y) -> Scope24/1, To Workspace/1

== system CAMFC2_01_WMR01/Data Bus /For matrix Plot13 ==
  epsilon : Inport
  MATLAB Function : MATLAB Function  TreatAsAtomicUnit=on
  Scope24 : Scope
  To Workspace : ToWorkspace  VariableName=epsilon2  SaveFormat=Structure With Time  SampleTime=-1
  wires:
  MATLAB Function/1(y) -> Scope24/1, To Workspace/1
  epsilon/1 -> MATLAB Function/1(u)

== system CAMFC2_01_WMR01/Data Bus /For matrix Plot14 ==
  epsilon : Inport
  MATLAB Function : MATLAB Function  TreatAsAtomicUnit=on
  Scope24 : Scope
  To Workspace : ToWorkspace  VariableName=epsilon3  SaveFormat=Structure With Time  SampleTime=-1
  wires:
  MATLAB Function/1(y) -> Scope24/1, To Workspace/1
  epsilon/1 -> MATLAB Function/1(u)

== system CAMFC2_01_WMR01/Data Bus /For matrix Plot15 ==
  epsilon : Inport
  MATLAB Function : MATLAB Function  TreatAsAtomicUnit=on
  Scope24 : Scope
  To Workspace : ToWorkspace  VariableName=epsilon4  SaveFormat=Structure With Time  SampleTime=-1
  wires:
  epsilon/1 -> MATLAB Function/1(u)
  MATLAB Function/1(y) -> Scope24/1, To Workspace/1

== system CAMFC2_01_WMR01/Data Bus /For matrix Plot2 ==
  P : Inport
  MATLAB Function : MATLAB Function  TreatAsAtomicUnit=on
  Scope24 : Scope
  To Workspace : ToWorkspace  VariableName=P3  SaveFormat=Structure With Time  SampleTime=-1
  wires:
  MATLAB Function/1(y) -> Scope24/1, To Workspace/1
  P/1 -> MATLAB Function/1(u)

== system CAMFC2_01_WMR01/Data Bus /For matrix Plot3 ==
  P : Inport
  MATLAB Function : MATLAB Function  TreatAsAtomicUnit=on
  Scope24 : Scope
  To Workspace : ToWorkspace  VariableName=P4  SaveFormat=Structure With Time  SampleTime=-1
  wires:
  P/1 -> MATLAB Function/1(u)
  MATLAB Function/1(y) -> Scope24/1, To Workspace/1

== system CAMFC2_01_WMR01/Data Bus /For matrix Plot4 ==
  A_hat : Inport
  MATLAB Function : MATLAB Function  TreatAsAtomicUnit=on
  Scope24 : Scope
  To Workspace : ToWorkspace  VariableName=A_hat1  SaveFormat=Structure With Time  SampleTime=-1
  wires:
  MATLAB Function/1(y) -> Scope24/1, To Workspace/1
  A_hat/1 -> MATLAB Function/1(u)

== system CAMFC2_01_WMR01/Data Bus /For matrix Plot5 ==
  A_hat : Inport
  MATLAB Function : MATLAB Function  TreatAsAtomicUnit=on
  Scope24 : Scope
  To Workspace : ToWorkspace  VariableName=A_hat2  SaveFormat=Structure With Time  SampleTime=-1
  wires:
  A_hat/1 -> MATLAB Function/1(u)
  MATLAB Function/1(y) -> Scope24/1, To Workspace/1

== system CAMFC2_01_WMR01/Data Bus /For matrix Plot6 ==
  A_hat : Inport
  MATLAB Function : MATLAB Function  TreatAsAtomicUnit=on
  Scope24 : Scope
  To Workspace : ToWorkspace  VariableName=A_hat3  SaveFormat=Structure With Time  SampleTime=-1
  wires:
  MATLAB Function/1(y) -> Scope24/1, To Workspace/1
  A_hat/1 -> MATLAB Function/1(u)

== system CAMFC2_01_WMR01/Data Bus /For matrix Plot7 ==
  A_hat : Inport
  MATLAB Function : MATLAB Function  TreatAsAtomicUnit=on
  Scope24 : Scope
  To Workspace : ToWorkspace  VariableName=A_hat4  SaveFormat=Structure With Time  SampleTime=-1
  wires:
  A_hat/1 -> MATLAB Function/1(u)
  MATLAB Function/1(y) -> Scope24/1, To Workspace/1

== system CAMFC2_01_WMR01/Data Bus /For matrix Plot8 ==
  T : Inport
  MATLAB Function : MATLAB Function  TreatAsAtomicUnit=on
  Scope24 : Scope
  To Workspace : ToWorkspace  VariableName=T1  SaveFormat=Structure With Time  SampleTime=-1
  wires:
  MATLAB Function/1(y) -> Scope24/1, To Workspace/1
  T/1 -> MATLAB Function/1(u)

== system CAMFC2_01_WMR01/Data Bus /For matrix Plot9 ==
  T : Inport
  MATLAB Function : MATLAB Function  TreatAsAtomicUnit=on
  Scope24 : Scope
  To Workspace : ToWorkspace  VariableName=T2  SaveFormat=Structure With Time  SampleTime=-1
  wires:
  T/1 -> MATLAB Function/1(u)
  MATLAB Function/1(y) -> Scope24/1, To Workspace/1

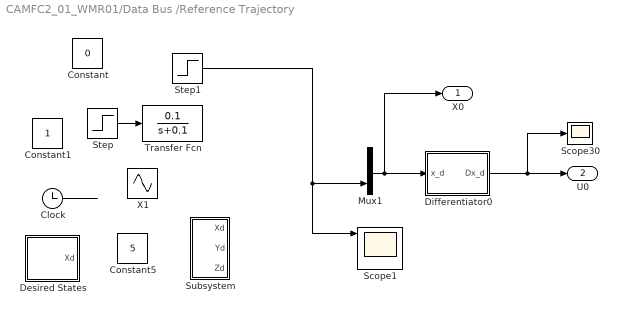
== system CAMFC2_01_WMR01/Data Bus /Reference Trajectory ==
  Clock : Clock
  Constant : Constant  Value=0
  Constant1 : Constant
  Constant5 : Constant  Value=5
  Desired States : Subsystem
  Differentiator0 : Subsystem
  Mux1 : Mux  Inputs=2
  Scope1 : Scope  NumInputPorts=3
  Scope30 : Scope
  Step : Step  Time=10  After=5  SampleTime=0
  Step1 : Step  Time=10  After=5  SampleTime=0
  Subsystem : Subsystem
  Transfer Fcn : TransferFcn  Numerator=[0.1]  Denominator=[1 0.1]
  X1 : Sin  Amplitude=5  Frequency=0.1  SampleTime=0
  X0 : Outport
  U0 : Outport  Port=2
  wires:
  Clock/1 -> ?
  Differentiator0/1(Dx_d) -> U0/1, Scope30/1
  ? -> Mux1/1
  Mux1/1 -> X0/1, Differentiator0/1(x_d)
  Step/1 -> Transfer Fcn/1
  Step1/1 -> Scope1/1, Mux1/2

== system CAMFC2_01_WMR01/Agent #1/Decenteralized Cooperaive Controller #1/Differentiator0 ==
  x_d : Inport
  Integrator : Integrator  InitialCondition=zeros(n0,1)
  Integrator1 : Integrator  InitialCondition=zeros(n0,1)
  Sliding differentiator : MATLAB Function  TreatAsAtomicUnit=on
  Sliding differentiator1 : MATLAB Function  TreatAsAtomicUnit=on
  Sum : Sum  Inputs=|-+
  Dx_d : Outport
  wires:
  Sliding differentiator/1(u) -> Integrator1/1, Dx_d/1
  Sliding differentiator1/1(Du1) -> Integrator/1
  Integrator/1 -> Sliding differentiator/1(u1)
  x_d/1 -> Sum/1
  Sum/1 -> Sliding differentiator/2(e), Sliding differentiator1/1(e)
  Integrator1/1 -> Sum/2

== system CAMFC2_01_WMR01/Agent #1/Decenteralized Cooperaive Controller #1/Differentiator1 ==
  x_d : Inport
  Integrator : Integrator  InitialCondition=zeros(n0,1)
  Integrator1 : Integrator  InitialCondition=zeros(n0,1)
  Sliding differentiator : MATLAB Function  TreatAsAtomicUnit=on
  Sliding differentiator1 : MATLAB Function  TreatAsAtomicUnit=on
  Sum : Sum  Inputs=|-+
  Dx_d : Outport
  wires:
  Integrator1/1 -> Sum/2
  Sum/1 -> Sliding differentiator1/1(e), Sliding differentiator/2(e)
  x_d/1 -> Sum/1
  Integrator/1 -> Sliding differentiator/1(u1)
  Sliding differentiator1/1(Du1) -> Integrator/1
  Sliding differentiator/1(u) -> Dx_d/1, Integrator1/1

== system CAMFC2_01_WMR01/Agent #1/Decenteralized Cooperaive Controller #1/Differentiator2 ==
  x_d : Inport
  Integrator : Integrator  InitialCondition=zeros(N+1,n)
  Integrator1 : Integrator  InitialCondition=zeros(N+1,n)
  Sliding differentiator : MATLAB Function  TreatAsAtomicUnit=on
  Sliding differentiator1 : MATLAB Function  TreatAsAtomicUnit=on
  Sum : Sum  Inputs=|-+
  Dx_d : Outport
  wires:
  Sliding differentiator/1(u) -> Integrator1/1, Dx_d/1
  Sliding differentiator1/1(Du1) -> Integrator/1
  Integrator/1 -> Sliding differentiator/1(u1)
  x_d/1 -> Sum/1
  Sum/1 -> Sliding differentiator/2(e), Sliding differentiator1/1(e)
  Integrator1/1 -> Sum/2

== system CAMFC2_01_WMR01/Agent #2/Decenteralized Cooperaive Controller #2/Differentiator0 ==
  x_d : Inport
  Integrator : Integrator  InitialCondition=zeros(n0,1)
  Integrator1 : Integrator  InitialCondition=zeros(n0,1)
  Sliding differentiator : MATLAB Function  TreatAsAtomicUnit=on
  Sliding differentiator1 : MATLAB Function  TreatAsAtomicUnit=on
  Sum : Sum  Inputs=|-+
  Dx_d : Outport
  wires:
  Sliding differentiator/1(u) -> Integrator1/1, Dx_d/1
  Sliding differentiator1/1(Du1) -> Integrator/1
  Integrator/1 -> Sliding differentiator/1(u1)
  x_d/1 -> Sum/1
  Sum/1 -> Sliding differentiator/2(e), Sliding differentiator1/1(e)
  Integrator1/1 -> Sum/2

== system CAMFC2_01_WMR01/Agent #2/Decenteralized Cooperaive Controller #2/Differentiator1 ==
  x_d : Inport
  Integrator : Integrator  InitialCondition=zeros(n0,1)
  Integrator1 : Integrator  InitialCondition=zeros(n0,1)
  Sliding differentiator : MATLAB Function  TreatAsAtomicUnit=on
  Sliding differentiator1 : MATLAB Function  TreatAsAtomicUnit=on
  Sum : Sum  Inputs=|-+
  Dx_d : Outport
  wires:
  Integrator1/1 -> Sum/2
  Sum/1 -> Sliding differentiator1/1(e), Sliding differentiator/2(e)
  x_d/1 -> Sum/1
  Integrator/1 -> Sliding differentiator/1(u1)
  Sliding differentiator1/1(Du1) -> Integrator/1
  Sliding differentiator/1(u) -> Dx_d/1, Integrator1/1

== system CAMFC2_01_WMR01/Agent #2/Decenteralized Cooperaive Controller #2/Differentiator2 ==
  x_d : Inport
  Integrator : Integrator  InitialCondition=zeros(N+1,n)
  Integrator1 : Integrator  InitialCondition=zeros(N+1,n)
  Sliding differentiator : MATLAB Function  TreatAsAtomicUnit=on
  Sliding differentiator1 : MATLAB Function  TreatAsAtomicUnit=on
  Sum : Sum  Inputs=|-+
  Dx_d : Outport
  wires:
  Sliding differentiator/1(u) -> Integrator1/1, Dx_d/1
  Sliding differentiator1/1(Du1) -> Integrator/1
  Integrator/1 -> Sliding differentiator/1(u1)
  x_d/1 -> Sum/1
  Sum/1 -> Sliding differentiator/2(e), Sliding differentiator1/1(e)
  Integrator1/1 -> Sum/2

== system CAMFC2_01_WMR01/Agent #3/Decenteralized Cooperaive Controller #3/Differentiator0 ==
  x_d : Inport
  Integrator : Integrator  InitialCondition=zeros(n0,1)
  Integrator1 : Integrator  InitialCondition=zeros(n0,1)
  Sliding differentiator : MATLAB Function  TreatAsAtomicUnit=on
  Sliding differentiator1 : MATLAB Function  TreatAsAtomicUnit=on
  Sum : Sum  Inputs=|-+
  Dx_d : Outport
  wires:
  Sliding differentiator/1(u) -> Integrator1/1, Dx_d/1
  Sliding differentiator1/1(Du1) -> Integrator/1
  Integrator/1 -> Sliding differentiator/1(u1)
  x_d/1 -> Sum/1
  Sum/1 -> Sliding differentiator/2(e), Sliding differentiator1/1(e)
  Integrator1/1 -> Sum/2

== system CAMFC2_01_WMR01/Agent #3/Decenteralized Cooperaive Controller #3/Differentiator1 ==
  x_d : Inport
  Integrator : Integrator  InitialCondition=zeros(n0,1)
  Integrator1 : Integrator  InitialCondition=zeros(n0,1)
  Sliding differentiator : MATLAB Function  TreatAsAtomicUnit=on
  Sliding differentiator1 : MATLAB Function  TreatAsAtomicUnit=on
  Sum : Sum  Inputs=|-+
  Dx_d : Outport
  wires:
  Integrator1/1 -> Sum/2
  Sum/1 -> Sliding differentiator1/1(e), Sliding differentiator/2(e)
  x_d/1 -> Sum/1
  Integrator/1 -> Sliding differentiator/1(u1)
  Sliding differentiator1/1(Du1) -> Integrator/1
  Sliding differentiator/1(u) -> Dx_d/1, Integrator1/1

== system CAMFC2_01_WMR01/Agent #3/Decenteralized Cooperaive Controller #3/Differentiator2 ==
  x_d : Inport
  Integrator : Integrator  InitialCondition=zeros(N+1,n)
  Integrator1 : Integrator  InitialCondition=zeros(N+1,n)
  Sliding differentiator : MATLAB Function  TreatAsAtomicUnit=on
  Sliding differentiator1 : MATLAB Function  TreatAsAtomicUnit=on
  Sum : Sum  Inputs=|-+
  Dx_d : Outport
  wires:
  Sliding differentiator/1(u) -> Integrator1/1, Dx_d/1
  Sliding differentiator1/1(Du1) -> Integrator/1
  Integrator/1 -> Sliding differentiator/1(u1)
  x_d/1 -> Sum/1
  Sum/1 -> Sliding differentiator/2(e), Sliding differentiator1/1(e)
  Integrator1/1 -> Sum/2

== system CAMFC2_01_WMR01/Agent #4/Decenteralized Cooperaive Controller #4/Differentiator0 ==
  x_d : Inport
  Integrator : Integrator  InitialCondition=zeros(n0,1)
  Integrator1 : Integrator  InitialCondition=zeros(n0,1)
  Sliding differentiator : MATLAB Function  TreatAsAtomicUnit=on
  Sliding differentiator1 : MATLAB Function  TreatAsAtomicUnit=on
  Sum : Sum  Inputs=|-+
  Dx_d : Outport
  wires:
  Sliding differentiator/1(u) -> Integrator1/1, Dx_d/1
  Sliding differentiator1/1(Du1) -> Integrator/1
  Integrator/1 -> Sliding differentiator/1(u1)
  x_d/1 -> Sum/1
  Sum/1 -> Sliding differentiator/2(e), Sliding differentiator1/1(e)
  Integrator1/1 -> Sum/2

== system CAMFC2_01_WMR01/Agent #4/Decenteralized Cooperaive Controller #4/Differentiator1 ==
  x_d : Inport
  Integrator : Integrator  InitialCondition=zeros(n0,1)
  Integrator1 : Integrator  InitialCondition=zeros(n0,1)
  Sliding differentiator : MATLAB Function  TreatAsAtomicUnit=on
  Sliding differentiator1 : MATLAB Function  TreatAsAtomicUnit=on
  Sum : Sum  Inputs=|-+
  Dx_d : Outport
  wires:
  Integrator1/1 -> Sum/2
  Sum/1 -> Sliding differentiator1/1(e), Sliding differentiator/2(e)
  x_d/1 -> Sum/1
  Integrator/1 -> Sliding differentiator/1(u1)
  Sliding differentiator1/1(Du1) -> Integrator/1
  Sliding differentiator/1(u) -> Dx_d/1, Integrator1/1

== system CAMFC2_01_WMR01/Agent #4/Decenteralized Cooperaive Controller #4/Differentiator2 ==
  x_d : Inport
  Integrator : Integrator  InitialCondition=zeros(N+1,n)
  Integrator1 : Integrator  InitialCondition=zeros(N+1,n)
  Sliding differentiator : MATLAB Function  TreatAsAtomicUnit=on
  Sliding differentiator1 : MATLAB Function  TreatAsAtomicUnit=on
  Sum : Sum  Inputs=|-+
  Dx_d : Outport
  wires:
  Sliding differentiator/1(u) -> Integrator1/1, Dx_d/1
  Sliding differentiator1/1(Du1) -> Integrator/1
  Integrator/1 -> Sliding differentiator/1(u1)
  x_d/1 -> Sum/1
  Sum/1 -> Sliding differentiator/2(e), Sliding differentiator1/1(e)
  Integrator1/1 -> Sum/2

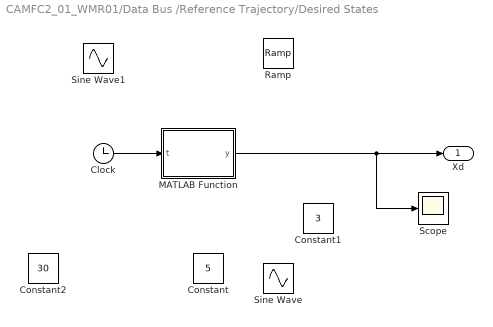
== system CAMFC2_01_WMR01/Data Bus /Reference Trajectory/Desired States ==
  Clock : Clock
  Constant : Constant  Value=5
  Constant1 : Constant  Value=3
  Constant2 : Constant  Value=30
  MATLAB Function : MATLAB Function  TreatAsAtomicUnit=on
  Ramp : simulink/Sources/Ramp  slope=5  start=0  X0=0
  Scope : Scope
  Sine Wave : Sin  Amplitude=2.5  Frequency=0.5  Phase=pi/2  SampleTime=0
  Sine Wave1 : Sin  Amplitude=5  Frequency=0.5  SampleTime=0
  Xd : Outport
  wires:
  Clock/1 -> MATLAB Function/1(t)
  MATLAB Function/1(y) -> Scope/1, Xd/1

== system CAMFC2_01_WMR01/Data Bus /Reference Trajectory/Differentiator0 ==
  x_d : Inport
  Integrator : Integrator  InitialCondition=zeros(n0,1)
  Integrator1 : Integrator  InitialCondition=zeros(n0,1)
  Sliding differentiator : MATLAB Function  TreatAsAtomicUnit=on
  Sliding differentiator1 : MATLAB Function  TreatAsAtomicUnit=on
  Sum : Sum  Inputs=|-+
  Dx_d : Outport
  wires:
  Sliding differentiator/1(u) -> Integrator1/1, Dx_d/1
  Sliding differentiator1/1(Du1) -> Integrator/1
  Integrator/1 -> Sliding differentiator/1(u1)
  x_d/1 -> Sum/1
  Sum/1 -> Sliding differentiator/2(e), Sliding differentiator1/1(e)
  Integrator1/1 -> Sum/2

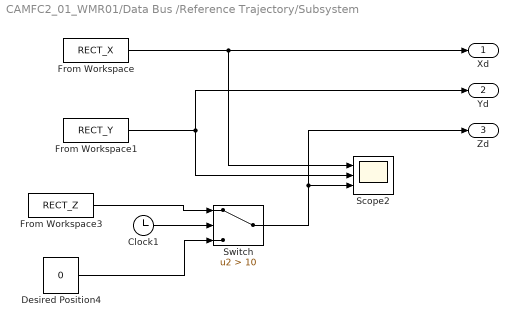
== system CAMFC2_01_WMR01/Data Bus /Reference Trajectory/Subsystem ==
  Clock1 : Clock
  Desired Position4 : Constant  Value=0  VectorParams1D=off
  From Workspace : FromWorkspace  VariableName=RECT_X  SampleTime=0
  From Workspace1 : FromWorkspace  VariableName=RECT_Y  SampleTime=0
  From Workspace3 : FromWorkspace  VariableName=RECT_Z  SampleTime=0
  Scope2 : Scope  NumInputPorts=3
  Switch : Switch  Criteria=u2 > Threshold  Threshold=10
  Xd : Outport
  Yd : Outport  Port=2
  Zd : Outport  Port=3
  wires:
  From Workspace/1 -> Xd/1, Scope2/1
  From Workspace1/1 -> Yd/1, Scope2/2
  Clock1/1 -> Switch/2
  Switch/1 -> Zd/1, Scope2/3
  From Workspace3/1 -> Switch/1
  Desired Position4/1 -> Switch/3

== matlab function CAMFC2_01_WMR01/Agent #1/Controller interpreter ==
  data: u output; U input
function u = fcn(U)

U1 = U(3);
U2 = U(4); 

u1 = 0.5 * (U1+U2);
u2 = 0.5 * (U1-U2);

u = [u1;u2];

end

== matlab function CAMFC2_01_WMR01/Agent #1/Decenteralized Cooperaive Controller #1/Adaptive Law A#1 ==
  data: Agent_Num input; A_hat input; gama2 parameter; rho2 parameter; T_i input; P_i input; DA_hat output; e_i input; H parameter; BN parameter; N parameter; n parameter; n0 parameter; z0 input; x input; ui input
function DA_hat = fcn(Agent_Num,A_hat,gama2,rho2,T_i,P_i,e_i,H,BN,N,n,n0,z0,x,ui)

%% 
z0_i = [z0;ui(1:n0)]; 

%%
vA_hat = diag(A_hat);

Sum = zeros(n,1);
for i=2:(N+1)
    Sum = Sum + (H(Agent_Num,(i-1)) * (2*x(((i-1)-1)*n+1:((i-1)*n),1)) - T_i(i,:)');
end
Sum = Sum + BN(Agent_Num,Agent_Num)*z0_i - e_i;
    
DvA_hat = -gama2*diag(Sum)*P_i * e_i - (rho2*gama2*vA_hat);

DA_hat = diag(DvA_hat);

end

== matlab function CAMFC2_01_WMR01/Agent #1/Decenteralized Cooperaive Controller #1/Adaptive Law g#1 ==
  data: Agent_Num input; g_hat input; gama1 parameter; rho1 parameter; P input; P_struct parameter; Dg_hat output; e input; H parameter; N parameter; n parameter
function Dg_hat = fcn(Agent_Num,g_hat,gama1,rho1,P,P_struct,e,H,N,n)

P_struct(1).data = P.p1;
P_struct(2).data = P.p2;
P_struct(3).data = P.p3;
P_struct(4).data = P.p4;

Sum = zeros(n,1);
for i=1:N  
    Sum = Sum + (H(i,Agent_Num) * P_struct(i).data * e((i-1)*n+1:(i*n),1)); %Adaptive law
end
    
Dg_hat = -gama1*Sum - (rho1*gama1*g_hat);

end

== matlab function CAMFC2_01_WMR01/Agent #1/Decenteralized Cooperaive Controller #1/Approx. U#1 ==
  data: Agent_Num input; q_i input; DT_i input; Approx_U_i output; B_pseudo_inverse parameter; A_hat_i input; x_i input; g_hat_i input
function Approx_U_i  = fcn(Agent_Num,q_i,DT_i,B_pseudo_inverse,A_hat_i,x_i,g_hat_i)

D_eta_0 = DT_i(1,:)';
D_eta_i = DT_i(Agent_Num,:)';

u0_i = q_i;

Approx_U_i = B_pseudo_inverse * (u0_i - A_hat_i * x_i - g_hat_i + D_eta_i - D_eta_0);

end
